simulink model "hw3_tustin_delay"  (R2015b)
settings: Solver=VariableStepAuto  StartTime=0.0  StopTime=10.0  RelTol=1e-3
values from neighbouring files (symbols this model uses):
  Td = 0.1    [hw3_spring16.m]    (also in hw4.m = Tu/8)
undefined symbols (not defined in the file or in its folder): Fdden, Fdnum, Gden, Gnum
settings Model: Creator=kjartan  LastModifiedBy=kjartan

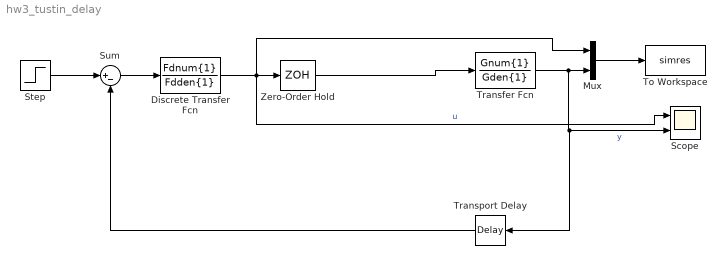
== system hw3_tustin_delay ==
  Discrete Transfer Fcn : DiscreteTransferFcn  Numerator=Fdnum{1}  Denominator=Fdden{1}  SampleTime=Td
  Mux : Mux  Inputs=2
  Scope : Scope  NumInputPorts=2
  Step : Step  SampleTime=0
  Sum : Sum  Inputs=|+-
  To Workspace : ToWorkspace  VariableName=simres  SaveFormat=Timeseries  SampleTime=-1
  Transfer Fcn : TransferFcn  Numerator=Gnum{1}  Denominator=Gden{1}
  Transport Delay : TransportDelay  DelayTime=Td
  Zero-Order Hold : ZeroOrderHold  SampleTime=Td
  wires:
  Mux/1 -> To Workspace/1
  Transfer Fcn/1 -> Transport Delay/1, Scope/2, Mux/2  "y"
  Step/1 -> Sum/1
  Sum/1 -> Discrete Transfer Fcn/1
  Discrete Transfer Fcn/1 -> Mux/1, Scope/1, Zero-Order Hold/1  "u"
  Transport Delay/1 -> Sum/2
  Zero-Order Hold/1 -> Transfer Fcn/1
